simulink model "simple_model"  (R2017a)
settings: Solver=VariableStepAuto  StartTime=0.0  StopTime=10.0  RelTol=1e-3
values from neighbouring files (symbols this model uses):
  x0 = 100    [validate_model.m]
undefined symbols (not defined in the file or in its folder): sys, terop
settings Model: Creator=brunolnetto  LastModifiedBy=brunolnetto

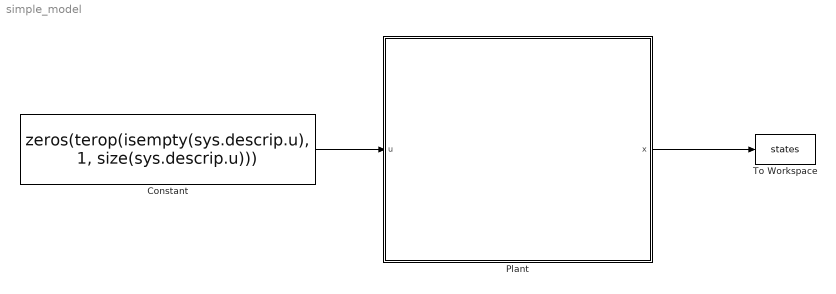
== system simple_model ==
  Constant : Constant  Value=zeros(terop(isempty(sys.descrip.u), 1, size(sys.descrip.u)))
  Plant : Subsystem
      mask Display: image('/home/brunolnetto/Pictures/vector_field.png');
  To Workspace : ToWorkspace  VariableName=states  SaveFormat=Structure With Time  SampleTime=-1
  wires:
  Plant/1(x) -> To Workspace/1
  Constant/1 -> Plant/1(u)

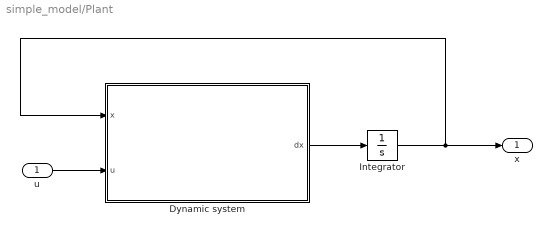
== system simple_model/Plant ==
  u : Inport
  Dynamic system : Subsystem
      mask Display: image('/home/brunolnetto/Pictures/dynamic_system.png');
  Integrator : Integrator  InitialCondition=x0
  x : Outport
  wires:
  Dynamic system/1(dx) -> Integrator/1
  u/1 -> Dynamic system/2(u)
  Integrator/1 -> Dynamic system/1(x), x/1

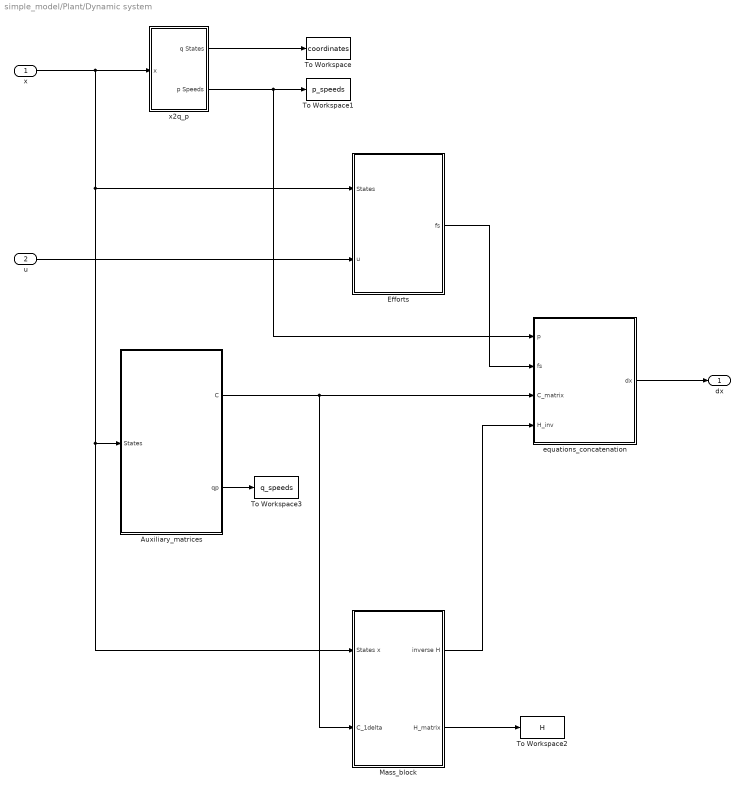
== system simple_model/Plant/Dynamic system ==
  x : Inport
  u : Inport  Port=2
  Auxiliary_matrices : Subsystem
  Efforts : Subsystem
  Mass_block : Subsystem
  To Workspace : ToWorkspace  VariableName=coordinates  SaveFormat=Structure With Time  SampleTime=-1
  To Workspace1 : ToWorkspace  VariableName=p_speeds  SaveFormat=Structure With Time  SampleTime=-1
  To Workspace2 : ToWorkspace  VariableName=H  SaveFormat=Structure With Time  SampleTime=-1
  To Workspace3 : ToWorkspace  VariableName=q_speeds  SaveFormat=Structure With Time  SampleTime=-1
  equations_concatenation : Subsystem
  x2q_p : Subsystem
  dx : Outport
  wires:
  Auxiliary_matrices/1(C) -> Mass_block/2("C_1delta  "), equations_concatenation/3(C_matrix)
  Auxiliary_matrices/2(qp) -> To Workspace3/1
  x2q_p/2(p Speeds) -> To Workspace1/1, equations_concatenation/1(p)
  x2q_p/1(q States) -> To Workspace/1
  Efforts/1(fs) -> equations_concatenation/2(fs)
  Mass_block/1(inverse H) -> equations_concatenation/4(H_inv)
  equations_concatenation/1(dx) -> dx/1
  u/1 -> Efforts/2(u)
  x/1 -> x2q_p/1(x), Efforts/1(States), Mass_block/1(States x), Auxiliary_matrices/1(States)
  Mass_block/2(H_matrix) -> To Workspace2/1

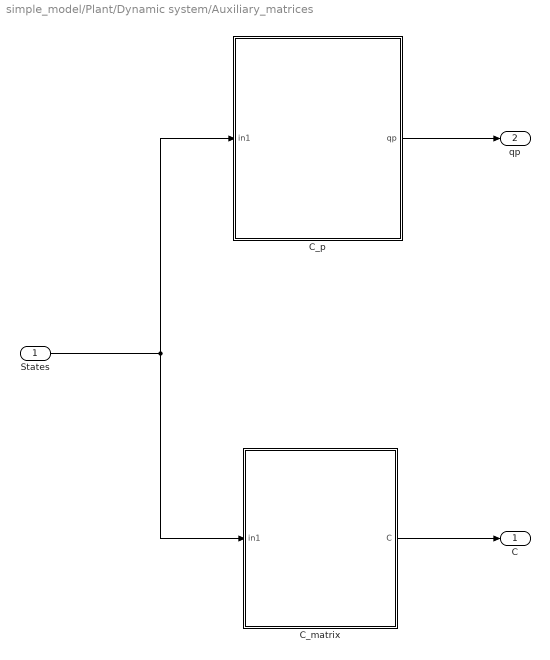
== system simple_model/Plant/Dynamic system/Auxiliary_matrices ==
  States : Inport
  C_matrix : MATLAB Function  TreatAsAtomicUnit=on
  C_p : MATLAB Function  TreatAsAtomicUnit=on
  C : Outport
  qp : Outport  Port=2
  wires:
  C_matrix/1(C) -> C/1
  States/1 -> C_p/1(in1), C_matrix/1(in1)
  C_p/1(qp) -> qp/1

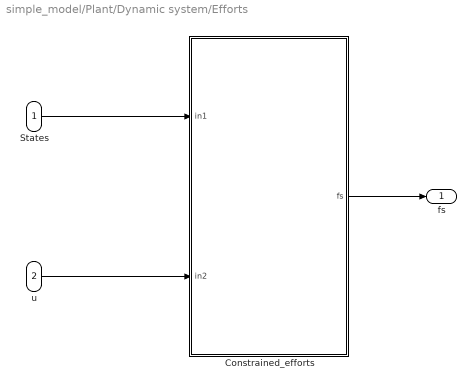
== system simple_model/Plant/Dynamic system/Efforts ==
  States : Inport
  u : Inport  Port=2
  Constrained_efforts : MATLAB Function  TreatAsAtomicUnit=on
  fs : Outport
  wires:
  States/1 -> Constrained_efforts/1(in1)
  u/1 -> Constrained_efforts/2(in2)
  Constrained_efforts/1(fs) -> fs/1

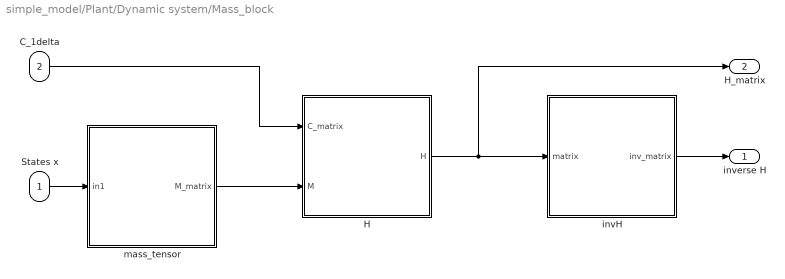
== system simple_model/Plant/Dynamic system/Mass_block ==
  States x : Inport
  "C_1delta  " : Inport  Port=2
  H : MATLAB Function  TreatAsAtomicUnit=on
  invH : MATLAB Function  TreatAsAtomicUnit=on
  mass_tensor : MATLAB Function  TreatAsAtomicUnit=on
  inverse H : Outport
  H_matrix : Outport  Port=2
  wires:
  States x/1 -> mass_tensor/1(in1)
  "C_1delta  "/1 -> H/1(C_matrix)
  invH/1(inv_matrix) -> inverse H/1
  H/1(H) -> invH/1(matrix), H_matrix/1
  mass_tensor/1(M_matrix) -> H/2(M)

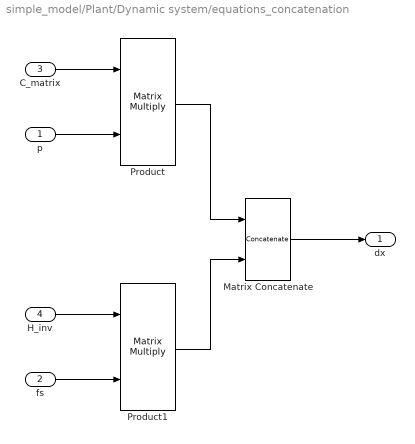
== system simple_model/Plant/Dynamic system/equations_concatenation ==
  p : Inport
  fs : Inport  Port=2
  C_matrix : Inport  Port=3
  H_inv : Inport  Port=4
  Matrix Concatenate : Concatenate  ConcatenateDimension=2
  Product : Product  Multiplication=Matrix(*)
  Product1 : Product  Multiplication=Matrix(*)
  dx : Outport
  wires:
  Product/1 -> Matrix Concatenate/1
  p/1 -> Product/2
  C_matrix/1 -> Product/1
  Product1/1 -> Matrix Concatenate/2
  H_inv/1 -> Product1/1
  fs/1 -> Product1/2
  Matrix Concatenate/1 -> dx/1

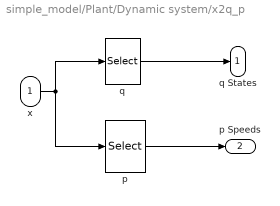
== system simple_model/Plant/Dynamic system/x2q_p ==
  x : Inport
  p : Selector  InputPortWidth=length(sys.kin.q) + length(sys.kin.p{end})  IndexOptions=Index vector (dialog)  Indices=(length(sys.kin.q))+1:(length(sys.kin.q) + length(sys.kin.p{end}))  OutputSizes=1
  q : Selector  InputPortWidth=length(sys.kin.q) + length(sys.kin.p{end})  IndexOptions=Index vector (dialog)  Indices=1:length(sys.kin.q)  OutputSizes=1
  q States : Outport
  p Speeds : Outport  Port=2
  wires:
  x/1 -> p/1, q/1
  q/1 -> q States/1
  p/1 -> p Speeds/1

== matlab function simple_model/Plant/Dynamic system/Mass_block/mass_tensor ==
  data: in1 input; M_matrix output
function M_matrix = Mass_matrix(in1)

%    This function was generated by the Symbolic Math Toolbox version 7.2.

%    21-Dec-2020 09:19:47



th1 = in1(4,:);

th2 = in1(5,:);

th3 = in1(6,:);

t2 = sin(th1);

t3 = sin(th2);

t4 = sin(th3);

M_matrix = reshape([2.11e2./5.0e2,0.0,0.0,0.0,0.0,0.0,0.0,2.11e2./5.0e2,0.0,0.0,0.0,0.0,0.0,0.0,t2.^2.*(-2.518133623269337e-7)-t3.^2.*2.518133623269337e-7-t4.^2.*2.518133623269337e-7+1.412783877342031e-2,0.0,0.0,0.0,0.0,0.0,0.0,0.0,0.0,0.0,0.0,0.0,0.0,0.0,0.0,0.0,0.0,0.0,0.0,0.0,0.0,0.0],[6,6]);

end

== matlab function simple_model/Plant/Dynamic system/Auxiliary_matrices/C_matrix ==
  data: in1 input; C output
function C = ConstraintMatrix(in1)

%    This function was generated by the Symbolic Math Toolbox version 7.2.

%    21-Dec-2020 09:19:47



th = in1(3,:);

t2 = pi.*(1.0./3.0);

t3 = t2+th;

C = reshape([sin(th).*(4.3e1./7.5e2),cos(th).*(-4.3e1./7.5e2),-4.3e1./3.75e2,1.0,0.0,0.0,cos(th+pi.*(1.0./6.0)).*(4.3e1./7.5e2),cos(-t2+th).*(4.3e1./7.5e2),-4.3e1./3.75e2,0.0,1.0,0.0,sin(t3).*(-4.3e1./7.5e2),cos(t3).*(4.3e1./7.5e2),-4.3e1./3.75e2,0.0,0.0,1.0],[6,3]);

end

== matlab function simple_model/Plant/Dynamic system/Efforts/Constrained_efforts ==
  data: in1 input; fs output; in2 input
function fs = ConstrainedEffort(in1,in2)

%    This function was generated by the Symbolic Math Toolbox version 7.2.

%    21-Dec-2020 09:19:47



p1 = in1(7,:);

p2 = in1(8,:);

p3 = in1(9,:);

tau1 = in2(1,:);

tau2 = in2(2,:);

tau3 = in2(3,:);

th1 = in1(4,:);

th2 = in1(5,:);

th3 = in1(6,:);

t2 = th1.*2.0;

t3 = sin(t2);

t4 = p1.*(4.3e1./3.75e2);

t5 = p2.*(4.3e1./3.75e2);

t6 = p3.*(4.3e1./3.75e2);

t7 = t4+t5+t6;

t8 = p1.*t3;

t9 = th2.*2.0;

t10 = sin(t9);

t11 = p2.*t10;

t12 = th3.*2.0;

t13 = sin(t12);

t14 = p3.*t13;

t15 = t8+t11+t14;

t16 = t7.*t15.*2.887459888015506e-8;

t17 = t7.^2;

fs = [t16+tau1-t3.*t17.*1.259066811634668e-7;t16+tau2-t10.*t17.*1.259066811634668e-7;t16+tau3-t13.*t17.*1.259066811634668e-7];

end

== matlab function simple_model/Plant/Dynamic system/Mass_block/H ==
  data: C_matrix input; H output; M input
function H = ConstrinedMassMatrix(C_matrix, M)
% MASSMATRIX
%    This function was generated by the Symbolic Math Toolbox version 7.2.
%    16-Oct-2020 11:55:07

    H = C_matrix'*M*C_matrix;
end

== matlab function simple_model/Plant/Dynamic system/Mass_block/invH ==
  data: matrix input; inv_matrix output
function inv_matrix = matrix_inverse(matrix)
% MASSMATRIX
%    This function was generated by the Symbolic Math Toolbox version 7.2.
%    16-Oct-2020 11:55:07

    inv_matrix = inv(matrix);
end

== matlab function simple_model/Plant/Dynamic system/Auxiliary_matrices/C_p ==
  data: in1 input; qp output
function qp = KinematicVector(in1)

%    This function was generated by the Symbolic Math Toolbox version 7.2.

%    21-Dec-2020 09:19:47



p1 = in1(7,:);

p2 = in1(8,:);

p3 = in1(9,:);

th = in1(3,:);

t2 = pi.*(1.0./3.0);

t3 = t2+th;

qp = [p2.*cos(th+pi.*(1.0./6.0)).*(4.3e1./7.5e2)-p3.*sin(t3).*(4.3e1./7.5e2)+p1.*sin(th).*(4.3e1./7.5e2);p3.*cos(t3).*(4.3e1./7.5e2)-p1.*cos(th).*(4.3e1./7.5e2)+p2.*cos(-t2+th).*(4.3e1./7.5e2);p1.*(-4.3e1./3.75e2)-p2.*(4.3e1./3.75e2)-p3.*(4.3e1./3.75e2);p1;p2;p3];

end
